simulink model "Buck_Boost_Converter"  (R2016a)
settings: Solver=VariableStepAuto  StartTime=0.0  StopTime=20  RelTol=1e-3
libraries: powerlib x13, re_lib x1, powerlib_meascontrol x1, dspstat3 x1
settings Model: Creator=Rangga  LastModifiedBy=Rangga

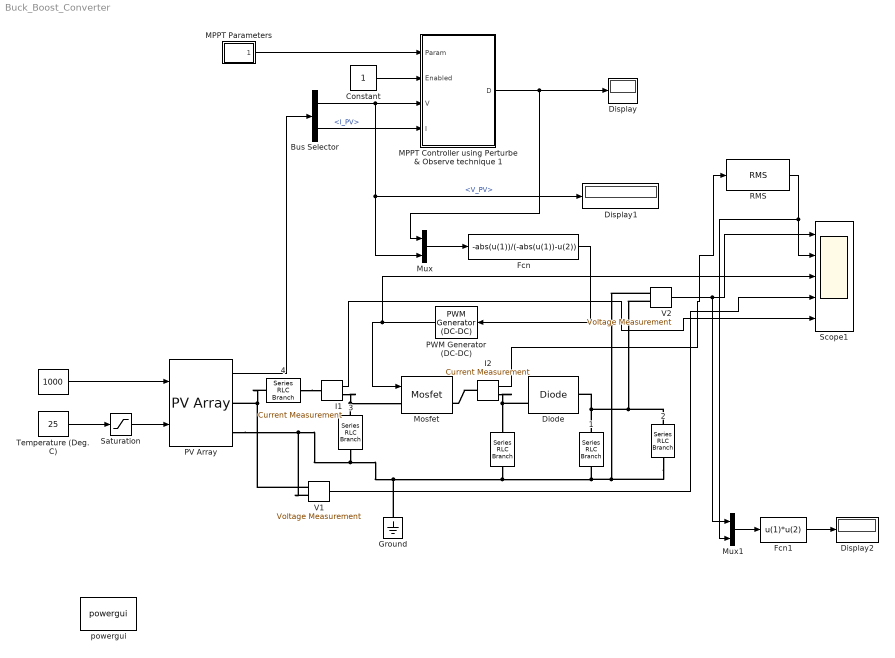
== system Buck_Boost_Converter ==
  " " : Constant  Value=1000
  " " : powerlib/Elements/Series RLC Branch  LConnTagsString=__new0  RConnTagsString=__new0  BranchType=L  Resistance=2  Inductance=2e-3  SetiL0=off  InitialCurrent=0  Capacitance=[]  Setx0=off  InitialVoltage=0  Measurements=None
  " 1" : powerlib/Elements/Series RLC Branch  LConnTagsString=__new0  RConnTagsString=__new0  BranchType=C  Resistance=2  Inductance=2e-3  SetiL0=off  InitialCurrent=0  Capacitance=0.01  Setx0=off  InitialVoltage=0  Measurements=None
  " 2" : powerlib/Elements/Series RLC Branch  LConnTagsString=__new0  RConnTagsString=__new0  BranchType=R  Resistance=5  Inductance=2e-3  SetiL0=off  InitialCurrent=0  Capacitance=0.01  Setx0=off  InitialVoltage=0  Measurements=None
  " 3" : powerlib/Elements/Series RLC Branch  LConnTagsString=__new0  RConnTagsString=__new0  BranchType=C  Resistance=3000e-6  Inductance=2e-3  SetiL0=off  InitialCurrent=0  Capacitance=10000e-6  Setx0=on  InitialVoltage=10  Measurements=None
  " 4" : powerlib/Elements/Series RLC Branch  LConnTagsString=__new0  RConnTagsString=__new0  BranchType=R  Resistance=1  Inductance=2e-3  SetiL0=off  InitialCurrent=0  Capacitance=0.01  Setx0=off  InitialVoltage=0  Measurements=None
  Bus Selector : BusSelector  OutputSignals=V_PV,I_PV
  Constant : Constant
  Diode : powerlib/Power Electronics/Diode  Ron=0.0001  Lon=0  Vf=0.8  IC=0  UseSnubber=off  Rs=0  Cs=0  Measurements=on
  Display : Display
  Display1 : Display
  Display2 : Display
  Fcn : Fcn  Expr=-abs(u(1))/(-abs(u(1))-u(2))
  Fcn1 : Fcn  Expr=u(1)*u(2)
  Ground : powerlib/Elements/Ground  LConnTagsString=a
  I1 : powerlib/Measurements/Current Measurement  Tag=PoWeRsYsTeMmEaSuReMeNt  PhasorSimulation=off  OutputType=Magnitude  PSBequivalent=0
  I2 : powerlib/Measurements/Current Measurement  Tag=PoWeRsYsTeMmEaSuReMeNt  PhasorSimulation=off  OutputType=Magnitude  PSBequivalent=0
  MPPT Parameters : Subsystem
  MPPT Controller using Perturbe & Observe technique 1 : MATLAB Function  TreatAsAtomicUnit=on
  Mosfet : powerlib/Power Electronics/Mosfet  Ron=0.1  Lon=0  Rd=0.01  Vfd=0  IC=0  Rs=1e5  Cs=inf  Measurements=on
  Mux : Mux  Inputs=2
  Mux1 : Mux  Inputs=2
  PV Array : re_lib/Solar/PV Array  Npar=1  Nser=1  PlotType=one module @ 25 deg.C & specified irradiances  S_vec=1000  Temp_C_vec=[ 45 25 100 ]  ModuleName=User-defined  PlotWhenSelected=off  Pm=99.981  Ncell=36  Voc=22.5  Isc=5.75  Vm=18.9  Im=5.29  beta_Voc_pc=-0.35  alpha_Isc_pc=0.06  beta_Voc=-0.07875  alpha_Isc=0.00345  IL=5.7591  I0=1.3543e-10  nI=0.99573  Rsh=93.7325  Rs=0.14801  BAL=on  Tc=1e-6  Tfilter=5e-5
      settings: AttributesFormatString=|
      | %<ModuleName>
      | %<Nser>-module string
      | %<Npar> parallel strings
  "PWM Generator (DC-DC) " : powerlib_meascontrol/Pulse & Signal Generators/PWM Generator (DC-DC)  Fsw=60*20  Ts=0
  RMS : dspstat3/RMS  run=on  reset_popup=None  InputProcessing=Columns as channels (frame based)  directionMode=Entire input  dimension=1
  Saturation : Saturate  UpperLimit=55  LowerLimit=5
  Scope1 : Scope  NumInputPorts=5
  Temperature (Deg. C) : Constant  Value=25
  V1 : powerlib/Measurements/Voltage Measurement  Tag=PoWeRsYsTeMmEaSuReMeNt  PhasorSimulation=off  OutputType=Magnitude  PSBequivalent=0
  V2 : powerlib/Measurements/Voltage Measurement  Tag=PoWeRsYsTeMmEaSuReMeNt  PhasorSimulation=off  OutputType=Magnitude  PSBequivalent=0
  powergui : powerlib/powergui  Priority=1  SimulationMode=Discrete  SolverType=Tustin/Backward Euler (TBE)  SampleTime=50e-6  frequency=60  SPID=on  DisableSnubberDevices=off  DisableRonSwitches=off  DisableVfSwitches=off  SwTol=0  DisplayEquations=off  Interpol=off  ExternalGateDelay=off  methode=off  Ts=10  FunctionMessages=off  echomessages=off  HookPort=off  EnableUseOfTLC=off  x0status=blocks  frequencyindice=0  Pbase=100e6  ErrMax=1e-4  Iterations=50  UnitsV=kV  UnitsW=MW  buscounter=0  RestoreLinks=warning  ResistiveCurrentMeasurement=off  Frange=[0:2:500]  Ylog=off  Xlog=on  ShowGrid=off  save=off  variable=ZData  structure=0  ZoomFFT=off  StartTime=0.0  cycles=1  DisplayStyle=1  fundamental=60  FreqAxis=off  MaxFrequency=1000  frequencyindicesteady=1  RmsSteady=1  display=off
  wires:
  MPPT Parameters/1(Param) -> MPPT Controller using Perturbe & Observe technique 1/1(Param)
  Constant/1 -> MPPT Controller using Perturbe & Observe technique 1/2(Enabled)
  MPPT Controller using Perturbe & Observe technique 1/1(D) -> Mux/1, Display/1
  " "/1 -> PV Array/1
  Temperature (Deg. C)/1 -> Saturation/1
  Saturation/1 -> PV Array/2
  PV Array/1 -> Bus Selector/1
  Bus Selector/1 -> MPPT Controller using Perturbe & Observe technique 1/3(V), Display1/1, Mux/2  "<V_PV>"
  Bus Selector/2 -> MPPT Controller using Perturbe & Observe technique 1/4(I)  "<I_PV>"
  Mux/1 -> Fcn/1
  Fcn/1 -> "PWM Generator (DC-DC) "/1
  "PWM Generator (DC-DC) "/1 -> Scope1/3, Mosfet/1
  I2/1 -> RMS/1
  V2/1 -> Mux1/1, Scope1/1
  I1/1 -> Scope1/5
  V1/1 -> Scope1/4
  Mux1/1 -> Fcn1/1
  Fcn1/1 -> Display2/1
  RMS/1 -> Mux1/2, Scope1/2
  connections:
  " 3"/LConn1 -- Mosfet/LConn1 -- I1/RConn1
  Diode/RConn1 -- " "/LConn1 -- I2/RConn1
  " 1"/LConn1 -- V2/LConn2 -- " 2"/LConn1 -- Diode/LConn1
  " 2"/RConn1 -- V2/LConn1 -- Ground/LConn1 -- V1/LConn2 -- PV Array/RConn2 -- " 3"/RConn1 -- " "/RConn1 -- " 1"/RConn1
  I2/LConn1 -- Mosfet/RConn1
  V1/LConn1 -- " 4"/RConn1 -- PV Array/RConn1
  " 4"/LConn1 -- I1/LConn1

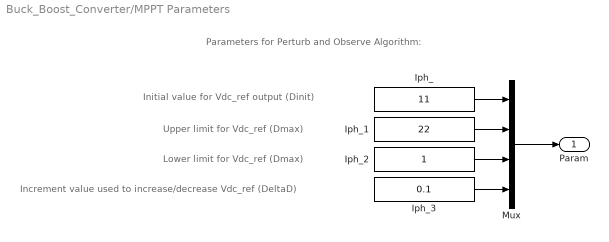
== system Buck_Boost_Converter/MPPT Parameters ==
  note: Upper limit for Vdc_ref (Dmax)
  note: Increment value used to increase/decrease Vdc_ref (DeltaD)
  note: Initial value for Vdc_ref output (Dinit)
  note: Lower limit for Vdc_ref (Dmax)
  note: Parameters for Perturb and Observe Algorithm:
  Iph_ : Constant  Value=11
  Iph_1 : Constant  Value=22
  Iph_2 : Constant
  Iph_3 : Constant  Value=0.1
  Mux : Mux
  Param : Outport
  wires:
  Iph_/1 -> Mux/1
  Iph_1/1 -> Mux/2
  Iph_2/1 -> Mux/3
  Iph_3/1 -> Mux/4
  Mux/1 -> Param/1

== matlab function Buck_Boost_Converter/MPPT Controller using Perturbe & Observe technique 1 ==
  settings: updateMethod=DISCRETE  sampleTime=Ts_Control
  data: Param input; Enabled input; V input; I input; D output
function D  = PandO(Param, Enabled, V, I)

% MPPT controller based on the Perturb & Observe algorithm.

% D output = Reference for DC link voltage (Vdc_ref) 
%
% Enabled input = 1 to enable the MPPT controller
% V input = PV array terminal voltage (V)
% I input = PV array current (A)
%
% Param input:
Dinit = Param(1);  %Initial value for Vdc_ref
Dmax = Param(2);   %Maximum value for Vdc_ref
Dmin = Param(3);   %Minimum value for Vdc_ref
deltaD = Param(4); %Increment value used to increase/decrease Vdc_ref
%  

persistent Vold Pold Dold;

dataType = 'double';

if isempty(Vold)
    Vold=0;
    Pold=0;
    Dold=Dinit;
end
P= V*I;
dV= V - Vold;
dP= P - Pold;

if dP ~= 0 & Enabled ~=0
    if dP < 0
        if dV < 0
            D = Dold + deltaD;
        else
            D = Dold - deltaD;
        end
    else
        if dV < 0
            D = Dold - deltaD;
        else
            D = Dold + deltaD;
        end    
    end
else D=Dold;
end

if D >= Dmax | D<= Dmin
    D=Dold;
end

Dold=D;
Vold=V;
Pold=P;
